simulink model "Back_emf_observer"  (Simulink 8.1)
settings: Solver=ode45  StartTime=0.0  StopTime=0.2  FixedStep=1e-6  MaxStep=1e-6  MinStep=0.5e-7  RelTol=1e-3
PreLoadFcn:
  | Parameter;
values from neighbouring files (symbols this model uses):
  Jm = 1e-4    (= 0.0001)    [Parameter.m]
  Kp = 1    [Parameter.m]
  Kw = 0.0573    [Parameter.m]
  La = 0.5e-3    (= 0.0005)    [Parameter.m]
  Ra = 0.25    [Parameter.m]
  Ti = La/Ra    (= 0.002)    [Parameter.m]
  Trated = Prated/Wrated    (= 0.238732414638)    [Parameter.m]
libraries: simulink x1
settings Model: Creator=a0131884  LastModifiedBy=a0131884
settings SolverCC: InitialStep=0.5e-7

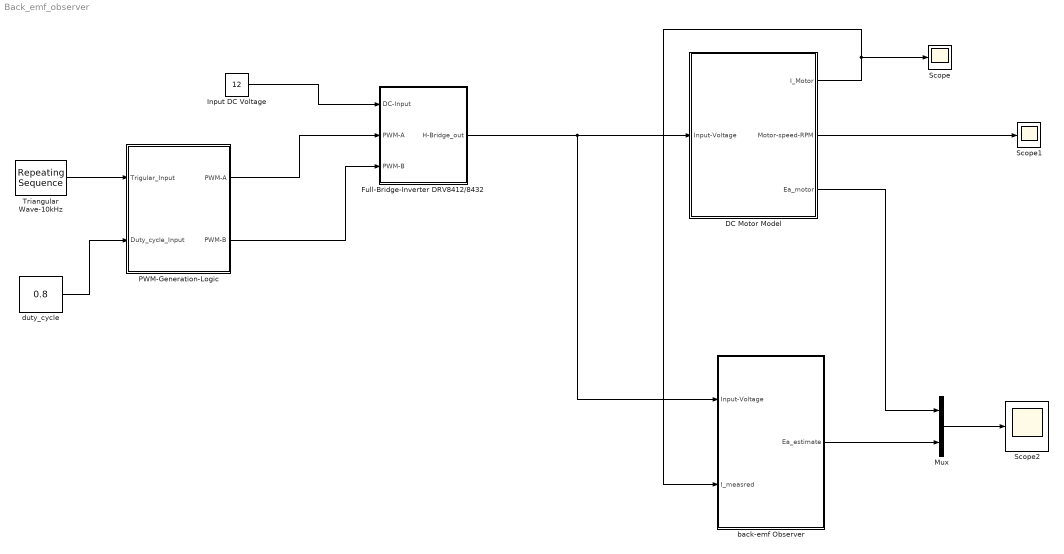
== system Back_emf_observer ==
  DC Motor Model : Subsystem
  Full-Bridge-Inverter DRV8412/8432 : Subsystem
  Input DC Voltage : Constant  Value=12
  Mux : Mux  Inputs=2
  PWM-Generation-Logic : Subsystem
  Scope : Scope
      settings: TimeRange=0.1  YMin=2.598470438397969  YMax=2.847579431295786
  Scope1 : Scope
      settings: TimeRange=0.35  YMin=0  YMax=1200
  Scope2 : Scope
      settings: TimeRange=0.2  YMin=-0.5  YMax=4.5  SaveName=ScopeData2
  Triangular Wave-10kHz : simulink/Sources/Repeating Sequence  rep_seq_t=[0 50e-6 100e-6]  rep_seq_y=[-1 1 -1]
  back-emf Observer : Subsystem
  duty_cycle : Constant  Value=0.8
  wires:
  DC Motor Model/2(Motor-speed-RPM) -> Scope1/1
  Input DC Voltage/1 -> Full-Bridge-Inverter DRV8412/8432/1(DC-Input)
  PWM-Generation-Logic/1(PWM-A) -> Full-Bridge-Inverter DRV8412/8432/2(PWM-A)
  PWM-Generation-Logic/2(PWM-B) -> Full-Bridge-Inverter DRV8412/8432/3(PWM-B)
  Triangular Wave-10kHz/1 -> PWM-Generation-Logic/1(Trigular_Input)
  duty_cycle/1 -> PWM-Generation-Logic/2(Duty_cycle_Input)
  DC Motor Model/1(I_Motor) -> Scope/1, back-emf Observer/2(I_measred)
  DC Motor Model/3(Ea_motor) -> Mux/1
  back-emf Observer/1(Ea_estimate) -> Mux/2
  Mux/1 -> Scope2/1
  Full-Bridge-Inverter DRV8412/8432/1(H-Bridge_out) -> back-emf Observer/1(Input-Voltage), DC Motor Model/1(Input-Voltage)

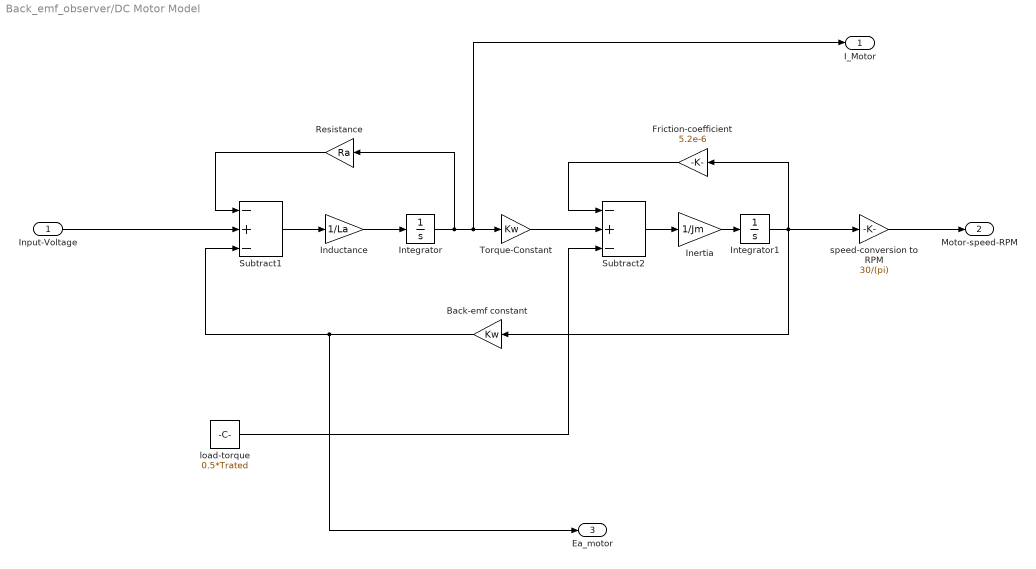
== system Back_emf_observer/DC Motor Model ==
  Input-Voltage : Inport
  Back-emf constant : Gain  Gain=Kw
  Friction-coefficient : Gain  Gain=5.2e-6
  Inductance : Gain  Gain=1/La
  Inertia : Gain  Gain=1/Jm
  Integrator : Integrator
  Integrator1 : Integrator
  Resistance : Gain  Gain=Ra
  Subtract1 : Sum  Inputs=-+-
  Subtract2 : Sum  Inputs=-+-
  Torque-Constant : Gain  Gain=Kw
  load-torque : Constant  Value=0.5*Trated
  speed-conversion to RPM : Gain  Gain=30/(pi)
  I_Motor : Outport
  Motor-speed-RPM : Outport  Port=2
  Ea_motor : Outport  Port=3
  wires:
  Subtract1/1 -> Inductance/1
  Inductance/1 -> Integrator/1
  Integrator/1 -> Resistance/1, I_Motor/1, Torque-Constant/1
  Resistance/1 -> Subtract1/1
  Torque-Constant/1 -> Subtract2/2
  Subtract2/1 -> Inertia/1
  Inertia/1 -> Integrator1/1
  Integrator1/1 -> Back-emf constant/1, speed-conversion to RPM/1, Friction-coefficient/1
  Friction-coefficient/1 -> Subtract2/1
  Back-emf constant/1 -> Ea_motor/1, Subtract1/3
  Input-Voltage/1 -> Subtract1/2
  load-torque/1 -> Subtract2/3
  speed-conversion to RPM/1 -> Motor-speed-RPM/1

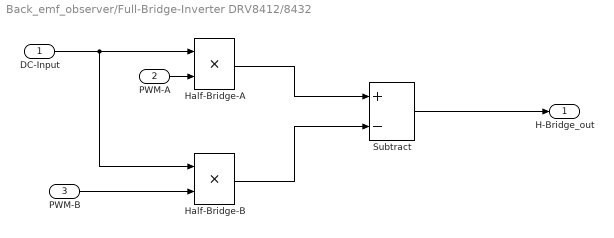
== system Back_emf_observer/Full-Bridge-Inverter DRV8412/8432 ==
  DC-Input : Inport
  PWM-A : Inport  Port=2
  PWM-B : Inport  Port=3
  Half-Bridge-A : Product  RndMeth=Zero
  Half-Bridge-B : Product  RndMeth=Zero
  Subtract : Sum  Inputs=+-
  H-Bridge_out : Outport
  wires:
  DC-Input/1 -> Half-Bridge-A/1, Half-Bridge-B/1
  PWM-A/1 -> Half-Bridge-A/2
  PWM-B/1 -> Half-Bridge-B/2
  Subtract/1 -> H-Bridge_out/1
  Half-Bridge-A/1 -> Subtract/1
  Half-Bridge-B/1 -> Subtract/2

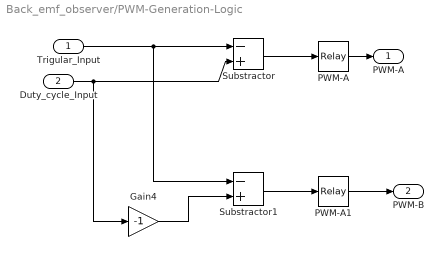
== system Back_emf_observer/PWM-Generation-Logic ==
  Trigular_Input : Inport
  Duty_cycle_Input : Inport  Port=2
  " PWM-A" : Relay  OnSwitchValue=0.000001  OffSwitchValue=-0.00001
  " PWM-A1" : Relay  OnSwitchValue=0.000001  OffSwitchValue=-0.00001
  Gain4 : Gain  Gain=-1  SaturateOnIntegerOverflow=on  OutDataTypeStr=Inherit: Same as input  ParamDataTypeStr=Inherit: Same as input
  Substractor : Sum  Inputs=-+
  Substractor1 : Sum  Inputs=-+
  PWM-A : Outport
  PWM-B : Outport  Port=2
  wires:
  Substractor/1 -> " PWM-A"/1
  Trigular_Input/1 -> Substractor/1, Substractor1/1
  " PWM-A"/1 -> PWM-A/1
  Duty_cycle_Input/1 -> Substractor/2, Gain4/1
  " PWM-A1"/1 -> PWM-B/1
  Substractor1/1 -> " PWM-A1"/1
  Gain4/1 -> Substractor1/2

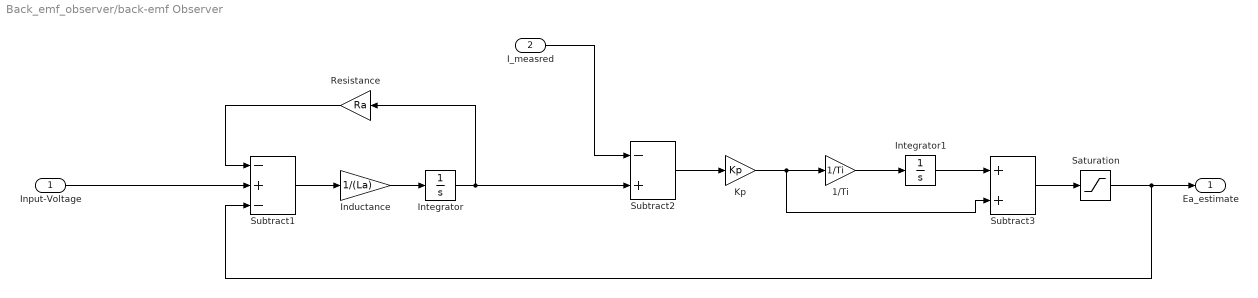
== system Back_emf_observer/back-emf Observer ==
  Input-Voltage : Inport
  I_measred : Inport  Port=2
  1/Ti : Gain  Gain=1/Ti
  Inductance : Gain  Gain=1/(La)
  Integrator : Integrator
  Integrator1 : Integrator  LimitOutput=on  UpperSaturationLimit=12  LowerSaturationLimit=-12
  Kp : Gain  Gain=Kp
  Resistance : Gain  Gain=Ra
  Saturation : Saturate  UpperLimit=12  LowerLimit=-12
  Subtract1 : Sum  Inputs=-+-
  Subtract2 : Sum  Inputs=-+
  Subtract3 : Sum
  Ea_estimate : Outport
  wires:
  Subtract1/1 -> Inductance/1
  Inductance/1 -> Integrator/1
  Integrator/1 -> Subtract2/2, Resistance/1
  Resistance/1 -> Subtract1/1
  Input-Voltage/1 -> Subtract1/2
  I_measred/1 -> Subtract2/1
  Subtract2/1 -> Kp/1
  Kp/1 -> Subtract3/2, 1/Ti/1
  1/Ti/1 -> Integrator1/1
  Integrator1/1 -> Subtract3/1
  Subtract3/1 -> Saturation/1
  Saturation/1 -> Subtract1/3, Ea_estimate/1
